simulink model "application"  (R2021b)
settings: Solver=FixedStepAuto  StartTime=0.0  StopTime=10.0  FixedStep=sampleTime  RelTol=1e-3
undefined symbols (not defined in the file or in its folder): AEMACE10_STBY, AEMACE8_STBY
libraries: simulink x10, EMACE_APP x6, AIL_STATE_MACHINE_LIB x2, AEMACE10_IN x1, AEMACE10_INSTRUMENTATION x1, AEMACE10_OUT x1, AEMACE8_IN x1, AEMACE8_INSTRUMENTATION x1, AEMACE8_OUT x1, SEMACE1_IN x1, SEMACE1_INSTRUMENTATION x1, SEMACE1_OUT x1
(part 1 of 2)
settings Model: Creator=ACH  LastModifiedBy=ACH

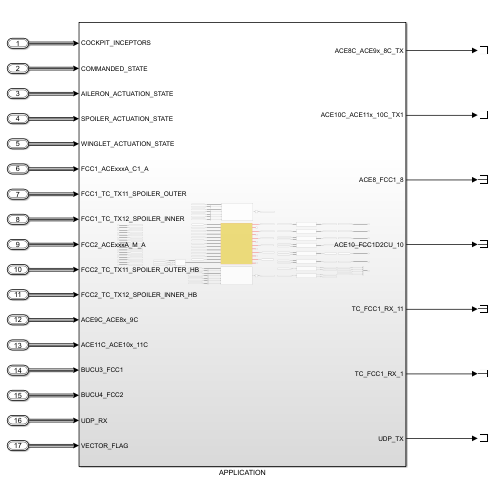
[thumbnail: Simulink's stored preview of the top-level diagram]
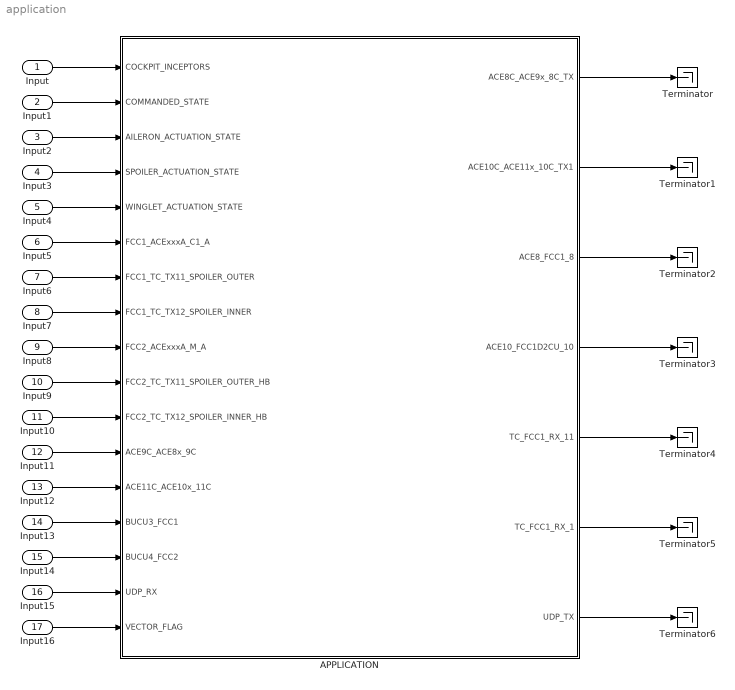
== system application ==
  Input : Inport  OutDataTypeStr=Bus: COCKPIT_INCEPTORS
  Input1 : Inport  Port=2  OutDataTypeStr=Bus: COMMANDED_STATE
  Input2 : Inport  Port=3  OutDataTypeStr=Bus: AILERON_ACTUATION_STATE
  Input3 : Inport  Port=4  OutDataTypeStr=Bus: SPOILER_ACTUATION_STATE
  Input4 : Inport  Port=5  OutDataTypeStr=Bus: WINGLET_ACTUATION_STATE
  Input5 : Inport  Port=6  OutDataTypeStr=Bus: FCC1_ACExxxA_C1_A
  Input6 : Inport  Port=7  OutDataTypeStr=Bus: FCC1_TC_TX_11_SPOILER_OUTER
  Input7 : Inport  Port=8  OutDataTypeStr=Bus: FCC1_TC_TX_12_SPOILER_INNER
  Input8 : Inport  Port=9  OutDataTypeStr=Bus: FCC2_ACExxxA_M_A
  Input9 : Inport  Port=10  OutDataTypeStr=Bus: FCC2_TC_TX_11_SPOILER_OUTER_HB
  Input10 : Inport  Port=11  OutDataTypeStr=Bus: FCC2_TC_TX_12_SPOILER_INNER_HB
  Input11 : Inport  Port=12  OutDataTypeStr=Bus: ACE9C_ACE8x_9C
  Input12 : Inport  Port=13  OutDataTypeStr=Bus: ACE11C_ACE10x_11C
  Input13 : Inport  Port=14  OutDataTypeStr=Bus: BUCU3_FCC1
  Input14 : Inport  Port=15  OutDataTypeStr=Bus: BUCU4_FCC2
  Input15 : Inport  Port=16  OutDataTypeStr=Bus: UDP_RX
  Input16 : Inport  Port=17  OutDataTypeStr=Bus: VECTOR_FLAG
  APPLICATION : Subsystem
  Terminator{,1..6} (7 alike) : Terminator
  wires:
  Input/1 -> APPLICATION/1(COCKPIT_INCEPTORS)
  Input1/1 -> APPLICATION/2(COMMANDED_STATE)
  Input2/1 -> APPLICATION/3(AILERON_ACTUATION_STATE)
  Input3/1 -> APPLICATION/4(SPOILER_ACTUATION_STATE)
  Input4/1 -> APPLICATION/5(WINGLET_ACTUATION_STATE)
  Input5/1 -> APPLICATION/6(FCC1_ACExxxA_C1_A)
  Input6/1 -> APPLICATION/7(FCC1_TC_TX11_SPOILER_OUTER)
  Input7/1 -> APPLICATION/8(FCC1_TC_TX12_SPOILER_INNER)
  Input8/1 -> APPLICATION/9(FCC2_ACExxxA_M_A)
  Input9/1 -> APPLICATION/10(FCC2_TC_TX11_SPOILER_OUTER_HB)
  Input10/1 -> APPLICATION/11(FCC2_TC_TX12_SPOILER_INNER_HB)
  Input11/1 -> APPLICATION/12(ACE9C_ACE8x_9C)
  Input12/1 -> APPLICATION/13(ACE11C_ACE10x_11C)
  Input13/1 -> APPLICATION/14(BUCU3_FCC1)
  Input14/1 -> APPLICATION/15(BUCU4_FCC2)
  Input15/1 -> APPLICATION/16(UDP_RX)
  Input16/1 -> APPLICATION/17(VECTOR_FLAG)
  APPLICATION/1(ACE8C_ACE9x_8C_TX) -> Terminator/1
  APPLICATION/2(ACE10C_ACE11x_10C_TX1) -> Terminator1/1
  APPLICATION/3(ACE8_FCC1_8) -> Terminator2/1
  APPLICATION/4(ACE10_FCC1D2CU_10) -> Terminator3/1
  APPLICATION/5(TC_FCC1_RX_11) -> Terminator4/1
  APPLICATION/6(TC_FCC1_RX_1) -> Terminator5/1
  APPLICATION/7(UDP_TX) -> Terminator6/1

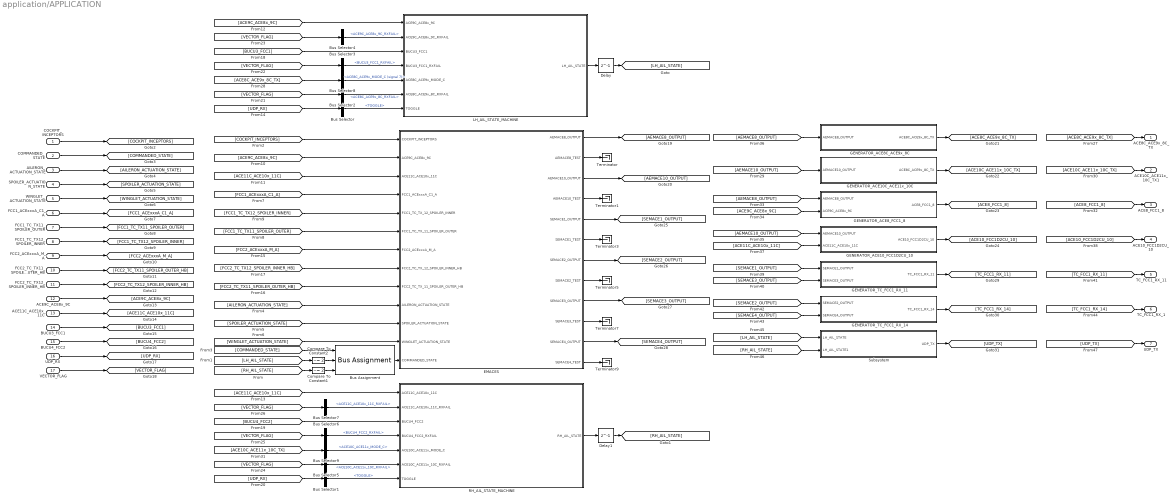
== system application/APPLICATION ==
  COCKPIT_INCEPTORS : Inport  OutDataTypeStr=Bus: COCKPIT_INCEPTORS
  COMMANDED_STATE : Inport  Port=2  OutDataTypeStr=Bus: COMMANDED_STATE
  AILERON_ACTUATION_STATE : Inport  Port=3  OutDataTypeStr=Bus: AILERON_ACTUATION_STATE
  SPOILER_ACTUATION_STATE : Inport  Port=4  OutDataTypeStr=Bus: SPOILER_ACTUATION_STATE
  WINGLET_ACTUATION_STATE : Inport  Port=5  OutDataTypeStr=Bus: WINGLET_ACTUATION_STATE
  FCC1_ACExxxA_C1_A : Inport  Port=6  OutDataTypeStr=Bus: FCC1_ACExxxA_C1_A
  FCC1_TC_TX11_SPOILER_OUTER : Inport  Port=7  OutDataTypeStr=Bus: FCC1_TC_TX_11_SPOILER_OUTER
  FCC1_TC_TX12_SPOILER_INNER : Inport  Port=8  OutDataTypeStr=Bus: FCC1_TC_TX_12_SPOILER_INNER
  FCC2_ACExxxA_M_A : Inport  Port=9  OutDataTypeStr=Bus: FCC2_ACExxxA_M_A
  FCC2_TC_TX11_SPOILER_OUTER_HB : Inport  Port=10  OutDataTypeStr=Bus: FCC2_TC_TX_11_SPOILER_OUTER_HB
  FCC2_TC_TX12_SPOILER_INNER_HB : Inport  Port=11  OutDataTypeStr=Bus: FCC2_TC_TX_12_SPOILER_INNER_HB
  ACE9C_ACE8x_9C : Inport  Port=12  OutDataTypeStr=Bus: ACE9C_ACE8x_9C
  ACE11C_ACE10x_11C : Inport  Port=13  OutDataTypeStr=Bus: ACE11C_ACE10x_11C
  BUCU3_FCC1 : Inport  Port=14  OutDataTypeStr=Bus: BUCU3_FCC1
  BUCU4_FCC2 : Inport  Port=15  OutDataTypeStr=Bus: BUCU4_FCC2
  UDP_RX : Inport  Port=16  OutDataTypeStr=Bus: UDP_RX
  VECTOR_FLAG : Inport  Port=17  OutDataTypeStr=Bus: VECTOR_FLAG
  Bus Assignment : BusAssignment  AssignedSignals=AEMACE8_STBY,AEMACE10_STBY
  Bus Selector : BusSelector  OutputSignals=TOGGLE
  Bus Selector1 : BusSelector  OutputSignals=TOGGLE
  Bus Selector2 : BusSelector  OutputSignals=ACE8C_ACE9x_8C_RXFAIL
  Bus Selector3 : BusSelector  OutputSignals=BUCU3_FCC1_RXFAIL
  Bus Selector4 : BusSelector  OutputSignals=ACE9C_ACE8x_9C_RXFAIL
  Bus Selector5 : BusSelector  OutputSignals=ACE10C_ACE11x_10C_RXFAIL
  Bus Selector6 : BusSelector  OutputSignals=BUCU4_FCC2_RXFAIL
  Bus Selector7 : BusSelector  OutputSignals=ACE11C_ACE10x_11C_RXFAIL
  Bus Selector8 : BusSelector  OutputSignals=ACE8C_ACE9x_MODE_C (signal 7)
  Bus Selector9 : BusSelector  OutputSignals=ACE10C_ACE11x_MODE_C
  Compare To Constant1 : simulink/Logic and Bit Operations/Compare To Constant  relop=~=  const=2  OutDataTypeStr=boolean
  Compare To Constant2 : simulink/Logic and Bit Operations/Compare To Constant  relop=~=  const=2  OutDataTypeStr=boolean
  Delay : Delay  DelayLength=1  InitialCondition=0
  Delay1 : Delay  DelayLength=1  InitialCondition=0
  EMACES : Subsystem
  GENERATOR_ACE10C_ACE11x_10C : Subsystem
  GENERATOR_ACE10_FCC1D2CU_10 : Subsystem
  GENERATOR_ACE8C_ACE9x_8C : Subsystem
  GENERATOR_ACE8_FCC1_8 : Subsystem
  GENERATOR_TC_FCC1_RX_11 : Subsystem
  GENERATOR_TC_FCC1_RX_14 : Subsystem
  LH_AIL_STATE_MACHINE : Subsystem
      settings: MinAlgLoopOccurrences=on
  RH_AIL_STATE_MACHINE : Subsystem
  Subsystem : Subsystem
  Terminator{,1,3,5,7,9} (6 alike) : Terminator
  ACE8C_ACE9x_8C_TX : Outport  OutDataTypeStr=Bus: ACE8C_ACE9x_8C
  ACE10C_ACE11x_10C_TX1 : Outport  Port=2  OutDataTypeStr=Bus: ACE10C_ACE11x_10C
  ACE8_FCC1_8 : Outport  Port=3  OutDataTypeStr=Bus: ACE8_FCC1_8
  ACE10_FCC1D2CU_10 : Outport  Port=4  OutDataTypeStr=Bus: ACE10_FCC1D2CU_10
  TC_FCC1_RX_11 : Outport  Port=5  OutDataTypeStr=Bus: TC_FCC1_RX_11
  TC_FCC1_RX_1 : Outport  Port=6  OutDataTypeStr=Bus: TC_FCC1_RX_14
  UDP_TX : Outport  Port=7  OutDataTypeStr=Bus: UDP_TX
  wires:
  [ACE11C_ACE10x_11C] -> EMACES/3(ACE11C_ACE10x_11C)
  [UDP_RX] -> Bus Selector1/1
  EMACES/9(SEMACE3_OUTPUT) -> [SEMACE3_OUTPUT]
  EMACES/12(SEMACE4_TEST) -> Terminator9/1
  Compare To Constant2/1 -> Bus Assignment/2
  RH_AIL_STATE_MACHINE/1(RH_AIL_STATE) -> Delay1/1
  [LH_AIL_STATE] -> Compare To Constant2/1
  [VECTOR_FLAG] -> Bus Selector4/1
  EMACES/11(SEMACE4_OUTPUT) -> [SEMACE4_OUTPUT]
  [AILERON_ACTUATION_STATE] -> EMACES/10(AILERON_ACTUATION_STATE)
  [ACE9C_ACE8x_9C] -> LH_AIL_STATE_MACHINE/1(ACE9C_ACE8x_9C)
  [ACE9C_ACE8x_9C] -> EMACES/2(ACE9C_ACE8x_9C)
  SPOILER_ACTUATION_STATE/1 -> [SPOILER_ACTUATION_STATE]
  [FCC2_ACExxxA_M_A] -> EMACES/7(FCC2_ACExxxA_M_A)
  Bus Selector1/1 -> RH_AIL_STATE_MACHINE/7(TOGGLE)  "<TOGGLE>"
  LH_AIL_STATE_MACHINE/1(LH_AIL_STATE) -> Delay/1
  Bus Selector2/1 -> LH_AIL_STATE_MACHINE/6(ACE8C_ACE9x_8C_RXFAIL)  "<ACE8C_ACE9x_8C_RXFAIL>"
  EMACES/6(SEMACE1_TEST) -> Terminator3/1
  EMACES/10(SEMACE3_TEST) -> Terminator7/1
  [WINGLET_ACTUATION_STATE] -> EMACES/12(WINGLET_ACTUATION_STATE)
  [FCC2_TC_TX11_SPOILER_OUTER_HB] -> EMACES/9(FCC2_TC_TX_11_SPOILER_OUTER_HB)
  [FCC1_ACExxxA_C1_A] -> EMACES/4(FCC1_ACExxxA_C1_A)
  [RH_AIL_STATE] -> Compare To Constant1/1
  WINGLET_ACTUATION_STATE/1 -> [WINGLET_ACTUATION_STATE]
  EMACES/5(SEMACE1_OUTPUT) -> [SEMACE1_OUTPUT]
  [SPOILER_ACTUATION_STATE] -> EMACES/11(SPOILER_ACTUATION_STATE)
  Bus Selector4/1 -> LH_AIL_STATE_MACHINE/2(ACE9C_ACE8x_9C_RXFAIL)  "<ACE9C_ACE8x_9C_RXFAIL>"
  BUCU3_FCC1/1 -> [BUCU3_FCC1]
  EMACES/2(AEMACE8_TEST) -> Terminator/1
  Bus Assignment/1 -> EMACES/13(COMMANDED_STATE)
  [COMMANDED_STATE] -> Bus Assignment/1
  FCC1_TC_TX11_SPOILER_OUTER/1 -> [FCC1_TC_TX11_SPOILER_OUTER]
  EMACES/4(AEMACE10_TEST) -> Terminator1/1
  EMACES/7(SEMACE2_OUTPUT) -> [SEMACE2_OUTPUT]
  [FCC1_TC_TX11_SPOILER_OUTER] -> EMACES/6(FCC1_TC_TX_11_SPOILER_OUTER)
  [UDP_RX] -> Bus Selector/1
  [VECTOR_FLAG] -> Bus Selector6/1
  Bus Selector7/1 -> RH_AIL_STATE_MACHINE/2(ACE11C_ACE10x_11C_RXFAIL)  "<ACE11C_ACE10x_11C_RXFAIL>"
  [VECTOR_FLAG] -> Bus Selector3/1
  Compare To Constant1/1 -> Bus Assignment/3
  Bus Selector3/1 -> LH_AIL_STATE_MACHINE/4(BUCU3_FCC1_RXFAIL)  "<BUCU3_FCC1_RXFAIL>"
  [VECTOR_FLAG] -> Bus Selector2/1
  [VECTOR_FLAG] -> Bus Selector5/1
  [FCC1_TC_TX12_SPOILER_INNER] -> EMACES/5(FCC1_TC_TX_12_SPOILER_INNER)
  Bus Selector/1 -> LH_AIL_STATE_MACHINE/7(TOGGLE)  "<TOGGLE>"
  Bus Selector5/1 -> RH_AIL_STATE_MACHINE/6(ACE10C_ACE11x_10C_RXFAIL)  "<ACE10C_ACE11x_10C_RXFAIL>"
  [BUCU4_FCC2] -> RH_AIL_STATE_MACHINE/3(BUCU4_FCC2)
  [ACE11C_ACE10x_11C] -> RH_AIL_STATE_MACHINE/1(ACE11C_ACE10x_11C)
  ACE11C_ACE10x_11C/1 -> [ACE11C_ACE10x_11C]
  EMACES/3(AEMACE10_OUTPUT) -> [AEMACE10_OUTPUT]
  [COCKPIT_INCEPTORS] -> EMACES/1(COCKPIT_INCEPTORS)
  Bus Selector6/1 -> RH_AIL_STATE_MACHINE/4(BUCU4_FCC2_RXFAIL)  "<BUCU4_FCC2_RXFAIL>"
  [FCC2_TC_TX12_SPOILER_INNER_HB] -> EMACES/8(FCC2_TC_TX_12_SPOILER_INNER_HB)
  EMACES/1(AEMACE8_OUTPUT) -> [AEMACE8_OUTPUT]
  FCC1_ACExxxA_C1_A/1 -> [FCC1_ACExxxA_C1_A]
  [VECTOR_FLAG] -> Bus Selector7/1
  [BUCU3_FCC1] -> LH_AIL_STATE_MACHINE/3(BUCU3_FCC1)
  EMACES/8(SEMACE2_TEST) -> Terminator5/1
  FCC2_ACExxxA_M_A/1 -> [FCC2_ACExxxA_M_A]
  COMMANDED_STATE/1 -> [COMMANDED_STATE]
  FCC2_TC_TX11_SPOILER_OUTER_HB/1 -> [FCC2_TC_TX11_SPOILER_OUTER_HB]
  ACE9C_ACE8x_9C/1 -> [ACE9C_ACE8x_9C]
  COCKPIT_INCEPTORS/1 -> [COCKPIT_INCEPTORS]
  UDP_RX/1 -> [UDP_RX]
  BUCU4_FCC2/1 -> [BUCU4_FCC2]
  FCC1_TC_TX12_SPOILER_INNER/1 -> [FCC1_TC_TX12_SPOILER_INNER]
  AILERON_ACTUATION_STATE/1 -> [AILERON_ACTUATION_STATE]
  FCC2_TC_TX12_SPOILER_INNER_HB/1 -> [FCC2_TC_TX12_SPOILER_INNER_HB]
  VECTOR_FLAG/1 -> [VECTOR_FLAG]
  Delay/1 -> [LH_AIL_STATE]
  Delay1/1 -> [RH_AIL_STATE]
  [ACE8C_ACE9x_8C_TX] -> ACE8C_ACE9x_8C_TX/1
  [AEMACE8_OUTPUT] -> GENERATOR_ACE8C_ACE9x_8C/1(AEMACE8_OUTPUT)
  GENERATOR_ACE8C_ACE9x_8C/1(ACE8C_ACE9x_8C_TX) -> [ACE8C_ACE9x_8C_TX]
  [ACE8C_ACE9x_8C_TX] -> Bus Selector8/1
  [AEMACE10_OUTPUT] -> GENERATOR_ACE10C_ACE11x_10C/1(AEMACE10_OUTPUT)
  GENERATOR_ACE10C_ACE11x_10C/1(ACE8C_ACE9x_8C_TX) -> [ACE10C_ACE11x_10C_TX]
  [ACE10C_ACE11x_10C_TX] -> ACE10C_ACE11x_10C_TX1/1
  [ACE10C_ACE11x_10C_TX] -> Bus Selector9/1
  Bus Selector9/1 -> RH_AIL_STATE_MACHINE/5(ACE10C_ACE11x_MODE_C)  "<ACE10C_ACE11x_MODE_C>"
  Bus Selector8/1 -> LH_AIL_STATE_MACHINE/5(ACE8C_ACE9x_MODE_C)  "<ACE8C_ACE9x_MODE_C (signal 7)>"
  GENERATOR_ACE8_FCC1_8/1(ACE8_FCC1_8) -> [ACE8_FCC1_8]
  [AEMACE8_OUTPUT] -> GENERATOR_ACE8_FCC1_8/1(AEMACE8_OUTPUT)
  [ACE8_FCC1_8] -> ACE8_FCC1_8/1
  [ACE9C_ACE8x_9C] -> GENERATOR_ACE8_FCC1_8/2(ACE9C_ACE8x_9C)
  [AEMACE10_OUTPUT] -> GENERATOR_ACE10_FCC1D2CU_10/1(AEMACE10_OUTPUT)
  [ACE11C_ACE10x_11C] -> GENERATOR_ACE10_FCC1D2CU_10/2(ACE11C_ACE10x_11C)
  GENERATOR_ACE10_FCC1D2CU_10/1(ACE10_FCC1D2CU_10) -> [ACE10_FCC1D2CU_10]
  [ACE10_FCC1D2CU_10] -> ACE10_FCC1D2CU_10/1
  [SEMACE1_OUTPUT] -> GENERATOR_TC_FCC1_RX_11/1(SEMACE1_OUTPUT)
  [SEMACE3_OUTPUT] -> GENERATOR_TC_FCC1_RX_11/2(SEMACE3_OUTPUT)
  GENERATOR_TC_FCC1_RX_11/1(TC_FCC1_RX_11) -> [TC_FCC1_RX_11]
  [TC_FCC1_RX_11] -> TC_FCC1_RX_11/1
  [TC_FCC1_RX_14] -> TC_FCC1_RX_1/1
  GENERATOR_TC_FCC1_RX_14/1(TC_FCC1_RX_14) -> [TC_FCC1_RX_14]
  [SEMACE4_OUTPUT] -> GENERATOR_TC_FCC1_RX_14/2(SEMACE4_OUTPUT)
  [SEMACE2_OUTPUT] -> GENERATOR_TC_FCC1_RX_14/1(SEMACE2_OUTPUT)
  [LH_AIL_STATE] -> Subsystem/1(LH_AIL_STATE)
  [RH_AIL_STATE] -> Subsystem/2(LH_AIL_STATE1)
  Subsystem/1(UDP_TX) -> [UDP_TX]
  [UDP_TX] -> UDP_TX/1

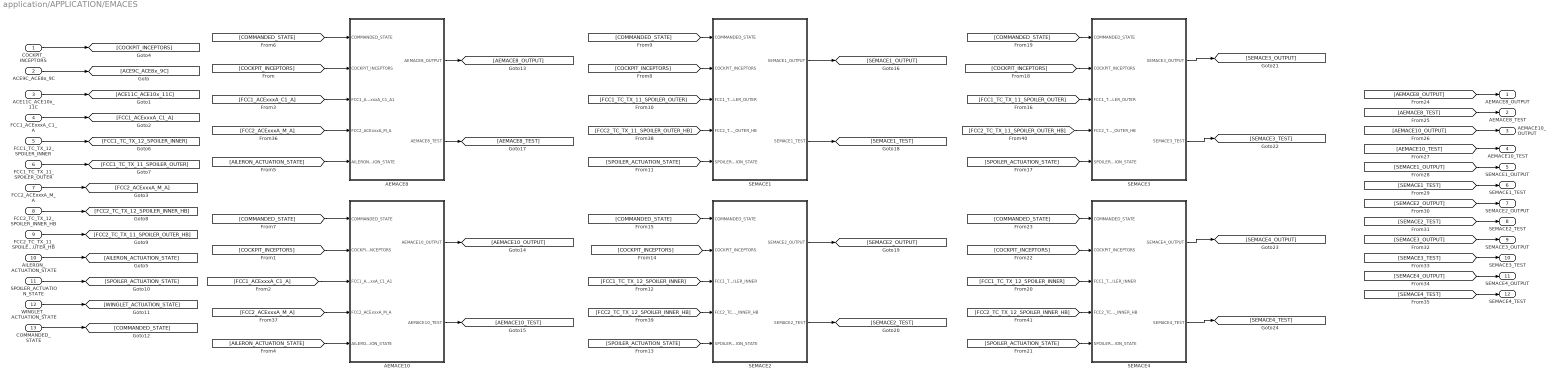
== system application/APPLICATION/EMACES ==
  COCKPIT_INCEPTORS : Inport  OutDataTypeStr=Bus: COCKPIT_INCEPTORS
  ACE9C_ACE8x_9C : Inport  Port=2  OutDataTypeStr=Bus: ACE9C_ACE8x_9C
  ACE11C_ACE10x_11C : Inport  Port=3  OutDataTypeStr=Bus: ACE11C_ACE10x_11C
  FCC1_ACExxxA_C1_A : Inport  Port=4  OutDataTypeStr=Bus: FCC1_ACExxxA_C1_A
  FCC1_TC_TX_12_SPOILER_INNER : Inport  Port=5  OutDataTypeStr=Bus: FCC1_TC_TX_12_SPOILER_INNER
  FCC1_TC_TX_11_SPOILER_OUTER : Inport  Port=6  OutDataTypeStr=Bus: FCC1_TC_TX_11_SPOILER_OUTER
  FCC2_ACExxxA_M_A : Inport  Port=7  OutDataTypeStr=Bus: FCC2_ACExxxA_M_A
  FCC2_TC_TX_12_SPOILER_INNER_HB : Inport  Port=8  OutDataTypeStr=Bus: FCC2_TC_TX_12_SPOILER_INNER_HB
  FCC2_TC_TX_11_SPOILER_OUTER_HB : Inport  Port=9  OutDataTypeStr=Bus: FCC2_TC_TX_11_SPOILER_OUTER_HB
  AILERON_ACTUATION_STATE : Inport  Port=10  OutDataTypeStr=Bus: AILERON_ACTUATION_STATE
  SPOILER_ACTUATION_STATE : Inport  Port=11  OutDataTypeStr=Bus: SPOILER_ACTUATION_STATE
  WINGLET_ACTUATION_STATE : Inport  Port=12  OutDataTypeStr=Bus: WINGLET_ACTUATION_STATE
  COMMANDED_STATE : Inport  Port=13  OutDataTypeStr=Bus: COMMANDED_STATE
  AEMACE10 : Subsystem
  AEMACE8 : Subsystem
  SEMACE1 : Subsystem
  SEMACE2 : Subsystem
  SEMACE3 : Subsystem
  SEMACE4 : Subsystem
  AEMACE8_OUTPUT : Outport  OutDataTypeStr=Bus: AEMACE8_OUTPUT
  AEMACE8_TEST : Outport  Port=2  OutDataTypeStr=Bus: AEMACE8_TEST
  AEMACE10_OUTPUT : Outport  Port=3  OutDataTypeStr=Bus: AEMACE10_OUTPUT
  AEMACE10_TEST : Outport  Port=4  OutDataTypeStr=Bus: AEMACE10_TEST
  SEMACE1_OUTPUT : Outport  Port=5  OutDataTypeStr=Bus: SEMACE1_OUTPUT
  SEMACE1_TEST : Outport  Port=6  OutDataTypeStr=Bus: SEMACE1_TEST
  SEMACE2_OUTPUT : Outport  Port=7  OutDataTypeStr=Bus: SEMACE3_OUTPUT
  SEMACE2_TEST : Outport  Port=8  OutDataTypeStr=Bus: SEMACE2_TEST
  SEMACE3_OUTPUT : Outport  Port=9  OutDataTypeStr=Bus: SEMACE3_OUTPUT
  SEMACE3_TEST : Outport  Port=10  OutDataTypeStr=Bus: SEMACE3_TEST
  SEMACE4_OUTPUT : Outport  Port=11  OutDataTypeStr=Bus: SEMACE4_OUTPUT
  SEMACE4_TEST : Outport  Port=12  OutDataTypeStr=Bus: SEMACE4_TEST
  wires:
  AEMACE8/1(AEMACE8_OUTPUT) -> [AEMACE8_OUTPUT]
  [SPOILER_ACTUATION_STATE] -> SEMACE4/5(SPOILER_ACTUATION_STATE)
  [AILERON_ACTUATION_STATE] -> AEMACE10/5(AILERON_ACTUATION_STATE)
  SEMACE2/1(SEMACE2_OUTPUT) -> [SEMACE2_OUTPUT]
  SEMACE4/2(SEMACE4_TEST) -> [SEMACE4_TEST]
  [COMMANDED_STATE] -> SEMACE1/1(COMMANDED_STATE)
  [FCC1_ACExxxA_C1_A] -> AEMACE8/3(FCC1_ACExxxA_C1_A1)
  AEMACE10/2(AEMACE10_TEST) -> [AEMACE10_TEST]
  [AEMACE8_OUTPUT] -> AEMACE8_OUTPUT/1
  SEMACE1/2(SEMACE1_TEST) -> [SEMACE1_TEST]
  AEMACE10/1(AEMACE10_OUTPUT) -> [AEMACE10_OUTPUT]
  [COMMANDED_STATE] -> AEMACE8/1(COMMANDED_STATE)
  SEMACE2/2(SEMACE2_TEST) -> [SEMACE2_TEST]
  [FCC1_TC_TX_11_SPOILER_OUTER] -> SEMACE1/3(FCC1_TC_TX_11_SPOILER_OUTER)
  ACE9C_ACE8x_9C/1 -> [ACE9C_ACE8x_9C]
  FCC1_TC_TX_11_SPOILER_OUTER/1 -> [FCC1_TC_TX_11_SPOILER_OUTER]
  [SPOILER_ACTUATION_STATE] -> SEMACE2/5(SPOILER_ACTUATION_STATE)
  [COMMANDED_STATE] -> SEMACE3/1(COMMANDED_STATE)
  AEMACE8/2(AEMACE8_TEST) -> [AEMACE8_TEST]
  [SEMACE3_OUTPUT] -> SEMACE3_OUTPUT/1
  [FCC1_ACExxxA_C1_A] -> AEMACE10/3(FCC1_ACExxxA_C1_A1)
  [AEMACE10_TEST] -> AEMACE10_TEST/1
  [COCKPIT_INCEPTORS] -> SEMACE1/2(COCKPIT_INCEPTORS)
  [AILERON_ACTUATION_STATE] -> AEMACE8/5(AILERON_ACTUATION_STATE)
  SEMACE1/1(SEMACE1_OUTPUT) -> [SEMACE1_OUTPUT]
  [COCKPIT_INCEPTORS] -> SEMACE2/2(COCKPIT_INCEPTORS)
  ACE11C_ACE10x_11C/1 -> [ACE11C_ACE10x_11C]
  [COCKPIT_INCEPTORS] -> SEMACE3/2(COCKPIT_INCEPTORS)
  [SEMACE1_OUTPUT] -> SEMACE1_OUTPUT/1
  [FCC1_TC_TX_12_SPOILER_INNER] -> SEMACE4/3(FCC1_TC_TX_12_SPOILER_INNER)
  FCC2_ACExxxA_M_A/1 -> [FCC2_ACExxxA_M_A]
  [COCKPIT_INCEPTORS] -> AEMACE8/2(COCKPIT_INCEPTORS)
  [COCKPIT_INCEPTORS] -> SEMACE4/2(COCKPIT_INCEPTORS)
  [AEMACE8_TEST] -> AEMACE8_TEST/1
  [FCC1_TC_TX_12_SPOILER_INNER] -> SEMACE2/3(FCC1_TC_TX_12_SPOILER_INNER)
  [SEMACE4_OUTPUT] -> SEMACE4_OUTPUT/1
  [COMMANDED_STATE] -> SEMACE2/1(COMMANDED_STATE)
  [FCC1_TC_TX_11_SPOILER_OUTER] -> SEMACE3/3(FCC1_TC_TX_11_SPOILER_OUTER)
  FCC1_ACExxxA_C1_A/1 -> [FCC1_ACExxxA_C1_A]
  [COMMANDED_STATE] -> SEMACE4/1(COMMANDED_STATE)
  [SEMACE1_TEST] -> SEMACE1_TEST/1
  SEMACE3/2(SEMACE3_TEST) -> [SEMACE3_TEST]
  SEMACE3/1(SEMACE3_OUTPUT) -> [SEMACE3_OUTPUT]
  [COMMANDED_STATE] -> AEMACE10/1(COMMANDED_STATE)
  COMMANDED_STATE/1 -> [COMMANDED_STATE]
  FCC1_TC_TX_12_SPOILER_INNER/1 -> [FCC1_TC_TX_12_SPOILER_INNER]
  [SPOILER_ACTUATION_STATE] -> SEMACE3/5(SPOILER_ACTUATION_STATE)
  [SPOILER_ACTUATION_STATE] -> SEMACE1/5(SPOILER_ACTUATION_STATE)
  SEMACE4/1(SEMACE4_OUTPUT) -> [SEMACE4_OUTPUT]
  [COCKPIT_INCEPTORS] -> AEMACE10/2(COCKPIT_INCEPTORS)
  [SEMACE2_OUTPUT] -> SEMACE2_OUTPUT/1
  [AEMACE10_OUTPUT] -> AEMACE10_OUTPUT/1
  AILERON_ACTUATION_STATE/1 -> [AILERON_ACTUATION_STATE]
  [SEMACE2_TEST] -> SEMACE2_TEST/1
  COCKPIT_INCEPTORS/1 -> [COCKPIT_INCEPTORS]
  FCC2_TC_TX_12_SPOILER_INNER_HB/1 -> [FCC2_TC_TX_12_SPOILER_INNER_HB]
  FCC2_TC_TX_11_SPOILER_OUTER_HB/1 -> [FCC2_TC_TX_11_SPOILER_OUTER_HB]
  WINGLET_ACTUATION_STATE/1 -> [WINGLET_ACTUATION_STATE]
  SPOILER_ACTUATION_STATE/1 -> [SPOILER_ACTUATION_STATE]
  [SEMACE3_TEST] -> SEMACE3_TEST/1
  [SEMACE4_TEST] -> SEMACE4_TEST/1
  [FCC2_ACExxxA_M_A] -> AEMACE8/4(FCC2_ACExxxA_M_A)
  [FCC2_ACExxxA_M_A] -> AEMACE10/4(FCC2_ACExxxA_M_A)
  [FCC2_TC_TX_11_SPOILER_OUTER_HB] -> SEMACE1/4(FCC2_TC_TX_11_SPOILER_OUTER_HB)
  [FCC2_TC_TX_12_SPOILER_INNER_HB] -> SEMACE2/4(FCC2_TC_TX_12_SPOILER_INNER_HB)
  [FCC2_TC_TX_11_SPOILER_OUTER_HB] -> SEMACE3/4(FCC2_TC_TX_11_SPOILER_OUTER_HB)
  [FCC2_TC_TX_12_SPOILER_INNER_HB] -> SEMACE4/4(FCC2_TC_TX_12_SPOILER_INNER_HB)

== system application/APPLICATION/GENERATOR_ACE10C_ACE11x_10C ==
  AEMACE10_OUTPUT : Inport  OutDataTypeStr=Bus: AEMACE10_OUTPUT
  Bus Creator : BusCreator  Inputs=17  OutDataTypeStr=Bus: ACE8C_ACE9x_8C
  Bus Selector8 : BusSelector  OutputSignals=AEMACE10_mode,AEMACE10_gearingAPP,AEMACE10_RAM_POS,AEMACE10_ROLL_POS,AEMACE10_SPD_SEL
  Cast{,2..10} (10 alike) : DataTypeConversion  OutDataTypeStr=boolean
  Cast1 : DataTypeConversion  OutDataTypeStr=uint8
  Cast11 : DataTypeConversion  OutDataTypeStr=single
  Constant{,1..11} (12 alike) : Constant  Value=0
  Delay{2..6} (5 alike) : Delay  DelayLength=1  InitialCondition=0
  ACE8C_ACE9x_8C_TX : Outport  OutDataTypeStr=Bus: ACE10C_ACE11x_10C
  wires:
  Bus Selector8/3 -> Delay4/1  "<AEMACE10_RAM_POS>"
  Bus Selector8/5 -> Delay6/1  "<AEMACE10_SPD_SEL>"
  Delay6/1 -> [ACE10C_ACE11x_SPD_C]
  AEMACE10_OUTPUT/1 -> Bus Selector8/1
  Delay5/1 -> [ACE10C_ACE11x_ROLL_POS_C]
  Constant7/1 -> Cast7/1
  Delay3/1 -> [ACE10C_ACE11x_GEARING_APPLIED]
  Cast10/1 -> Bus Creator/16
  Constant3/1 -> Cast3/1
  Cast11/1 -> Bus Creator/14
  [ACE10C_ACE11x_ROLL_POS_C] -> Bus Creator/9  "ACE10C_ACE11x_ROLL_POS_C"
  Cast5/1 -> Bus Creator/10
  [ACE10C_ACE11x_SPD_C] -> Bus Creator/17  "ACE10C_ACE11x_SPD_C"
  Constant8/1 -> Cast8/1
  Constant2/1 -> Cast2/1
  Bus Selector8/2 -> Delay3/1  "<AEMACE10_gearingAPP>"
  Cast3/1 -> Bus Creator/5
  Constant1/1 -> Cast1/1
  Constant5/1 -> Cast5/1
  Constant6/1 -> Cast6/1
  Bus Creator/1 -> ACE8C_ACE9x_8C_TX/1
  Cast1/1 -> Bus Creator/3
  Constant10/1 -> Cast10/1
  Delay2/1 -> [ACE10C_ACE11x_MODE_C]
  Cast6/1 -> Bus Creator/11
  Delay4/1 -> [ACE10C_ACE11x_RAM_POS_C]
  Cast8/1 -> Bus Creator/13
  Bus Selector8/4 -> Delay5/1  "<AEMACE10_ROLL_POS>"
  Constant11/1 -> Cast11/1
  Bus Selector8/1 -> Delay2/1  "<AEMACE10_mode>"
  Cast9/1 -> Bus Creator/15
  [ACE10C_ACE11x_GEARING_APPLIED] -> Bus Creator/1  "ACE10C_ACE11x_GEARING_APPLIED"
  Cast7/1 -> Bus Creator/12
  [ACE10C_ACE11x_RAM_POS_C] -> Bus Creator/6  "ACE10C_ACE11x_RAM_POS_C"
  Constant9/1 -> Cast9/1
  Constant/1 -> Cast/1
  Cast4/1 -> Bus Creator/8
  [ACE10C_ACE11x_MODE_C] -> Bus Creator/7  "ACE10C_ACE11x_MODE_C"
  Constant4/1 -> Cast4/1
  Cast2/1 -> Bus Creator/4
  Cast/1 -> Bus Creator/2  "ACE10C_ACE11x_GEARING_APP_F_C"

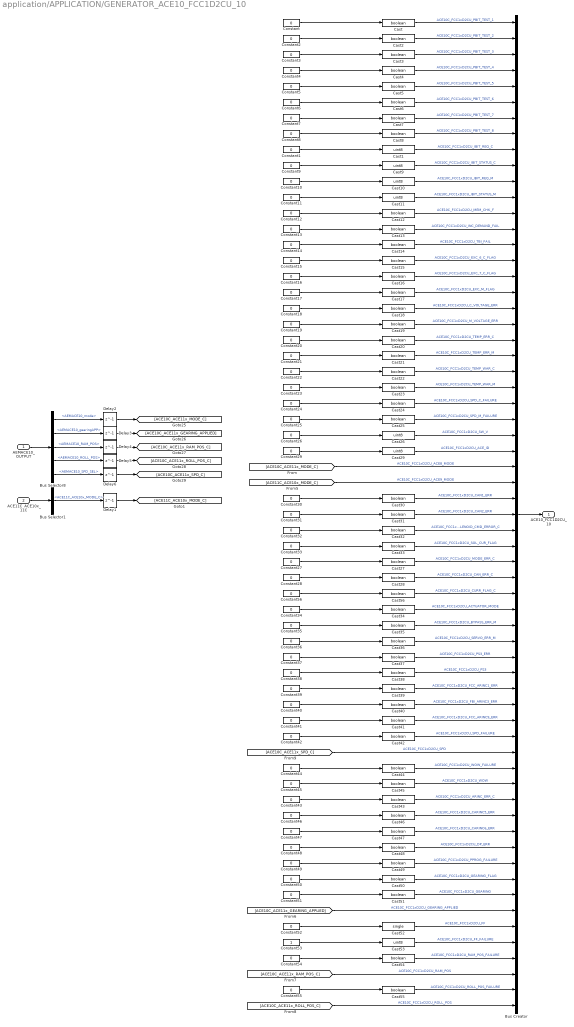
== system application/APPLICATION/GENERATOR_ACE10_FCC1D2CU_10 ==
  AEMACE10_OUTPUT : Inport  OutDataTypeStr=Bus: AEMACE10_OUTPUT
  ACE11C_ACE10x_11C : Inport  Port=2  OutDataTypeStr=Bus: ACE11C_ACE10x_11C
  Bus Creator : BusCreator  Inputs=63  OutDataTypeStr=Bus: ACE8_FCC1_8
  Bus Selector1 : BusSelector  OutputSignals=ACE11C_ACE10x_MODE_C
  Bus Selector8 : BusSelector  OutputSignals=AEMACE10_mode,AEMACE10_gearingAPP,AEMACE10_RAM_POS,AEMACE10_ROLL_POS,AEMACE10_SPD_SEL
  Cast{,2..8,12..25,27..28,30..51,54..56} (49 alike) : DataTypeConversion  OutDataTypeStr=boolean
  Cast{1,9..11,26,29,53} (7 alike) : DataTypeConversion  OutDataTypeStr=uint8
  Cast52 : DataTypeConversion  OutDataTypeStr=single
  Constant{,1..52,54..56} (56 alike) : Constant  Value=0
  Constant53 : Constant
  Delay{1..6} (6 alike) : Delay  DelayLength=1  InitialCondition=0
  ACE10_FCC1D2CU_10 : Outport  OutDataTypeStr=Bus: ACE10_FCC1D2CU_10
  wires:
  Cast56/1 -> Bus Creator/37  "ACE10C_FCC1xD2CU_CURR_FLAG_C"
  Constant56/1 -> Cast56/1
  Cast28/1 -> Bus Creator/36  "ACE10C_FCC1xD2CU_CAN_ERR_C"
  Constant28/1 -> Cast28/1
  Cast27/1 -> Bus Creator/35  "ACE10C_FCC1xD2CU_MODE_ERR_C"
  Constant27/1 -> Cast27/1
  Cast34/1 -> Bus Creator/38  "ACE10C_FCC1xD2CU_ACTUATOR_MODE"
  Cast36/1 -> Bus Creator/40  "ACE10C_FCC1xD2CU_SERVO_ERR_M"
  Constant34/1 -> Cast34/1
  Cast35/1 -> Bus Creator/39  "ACE10C_FCC1xD2CU_BYPASS_ERR_M"
  Constant36/1 -> Cast36/1
  Constant35/1 -> Cast35/1
  Constant39/1 -> Cast39/1
  Cast39/1 -> Bus Creator/43  "ACE10C_FCC1xD2CU_FCC_ARINC1_ERR"
  Cast37/1 -> Bus Creator/41  "ACE10C_FCC1xD2CU_PS3_ERR"
  Cast41/1 -> Bus Creator/45  "ACE10C_FCC1xD2CU_FCC_ARINC9_ERR"
  Constant38/1 -> Cast38/1
  Constant37/1 -> Cast37/1
  Cast38/1 -> Bus Creator/42  "ACE10C_FCC1xD2CU_PS3"
  Constant40/1 -> Cast40/1
  Constant41/1 -> Cast41/1
  Cast40/1 -> Bus Creator/44  "ACE10C_FCC1xD2CU_FBI_ARINC3_ERR"
  Cast44/1 -> Bus Creator/48  "ACE10C_FCC1xD2CU_WOW_FAILURE"
  Cast45/1 -> Bus Creator/49  "ACE10C_FCC1xD2CU_WOW"
  [ACE10C_ACE11x_SPD_C] -> Bus Creator/47  "ACE10C_FCC1xD2CU_SPD"
  Constant44/1 -> Cast44/1
  Cast42/1 -> Bus Creator/46  "ACE10C_FCC1xD2CU_SPD_FAILURE"
  Constant45/1 -> Cast45/1
  Constant42/1 -> Cast42/1
  Cast46/1 -> Bus Creator/51  "ACE10C_FCC1xD2CU_CARINC5_ERR"
  Cast48/1 -> Bus Creator/53  "ACE10C_FCC1xD2CU_DP_ERR"
  Constant48/1 -> Cast48/1
  Constant46/1 -> Cast46/1
  Cast43/1 -> Bus Creator/50  "ACE10C_FCC1xD2CU_ARINC_ERR_C"
  Constant43/1 -> Cast43/1
  Constant47/1 -> Cast47/1
  Cast47/1 -> Bus Creator/52  "ACE10C_FCC1xD2CU_CARINC6_ERR"
  Cast50/1 -> Bus Creator/55  "ACE10C_FCC1xD2CU_GEARING_FLAG"
  Cast51/1 -> Bus Creator/56  "ACE10C_FCC1xD2CU_GEARING"
  Cast49/1 -> Bus Creator/54  "ACE10C_FCC1xD2CU_PPROG_FAILURE"
  Constant50/1 -> Cast50/1
  Constant51/1 -> Cast51/1
  Constant49/1 -> Cast49/1
  [ACE10C_ACE11x_GEARING_APPLIED] -> Bus Creator/57  "ACE10C_FCC1xD2CU_GEARING_APPLIED"
  Constant53/1 -> Cast53/1
  Constant52/1 -> Cast52/1
  Cast52/1 -> Bus Creator/58  "ACE10C_FCC1xD2CU_FF"
  Cast53/1 -> Bus Creator/59  "ACE10C_FCC1xD2CU_FF_FAILURE"
  Cast54/1 -> Bus Creator/60  "ACE10C_FCC1xD2CU_RAM_POS_FAILURE"
  Constant54/1 -> Cast54/1
  [ACE10C_ACE11x_RAM_POS_C] -> Bus Creator/61  "ACE10C_FCC1xD2CU_RAM_POS"
  Constant55/1 -> Cast55/1
  Cast55/1 -> Bus Creator/62  "ACE10C_FCC1xD2CU_ROLL_POS_FAILURE"
  [ACE10C_ACE11x_ROLL_POS_C] -> Bus Creator/63  "ACE10C_FCC1xD2CU_ROLL_POS"
  [ACE11C_ACE10x_MODE_C] -> Bus Creator/30  "ACE10C_FCC1xD2CU_ACE9_MODE"
  Delay1/1 -> [ACE11C_ACE10x_MODE_C]
  Bus Selector1/1 -> Delay1/1  "<ACE11C_ACE10x_MODE_C>"
  ACE11C_ACE10x_11C/1 -> Bus Selector1/1
  Constant33/1 -> Cast33/1
  Cast33/1 -> Bus Creator/34  "ACE10C_FCC1xD2CU_SOL_CUR_FLAG"
  Cast32/1 -> Bus Creator/33  "ACE10C_FCC1xD2CU_SOLENOID_CMD_ERROR_C"
  Constant32/1 -> Cast32/1
  Constant31/1 -> Cast31/1
  Cast31/1 -> Bus Creator/32  "ACE10C_FCC1xD2CU_CAN2_ERR"
  Cast30/1 -> Bus Creator/31  "ACE10C_FCC1xD2CU_CAN1_ERR"
  Constant30/1 -> Cast30/1
  Cast26/1 -> Bus Creator/27  "ACE10C_FCC1xD2CU_SW_V"
  Constant26/1 -> Cast26/1
  Constant29/1 -> Cast29/1
  Cast29/1 -> Bus Creator/28  "ACE10C_FCC1xD2CU_ACE_ID"
  [ACE10C_ACE11x_MODE_C] -> Bus Creator/29  "ACE10C_FCC1xD2CU_ACE8_MODE"
  Constant25/1 -> Cast25/1
  Cast25/1 -> Bus Creator/26  "ACE10C_FCC1xD2CU_SPD_M_FAILURE"
  Cast24/1 -> Bus Creator/25  "ACE10C_FCC1xD2CU_SPD_C_FAILURE"
  Constant24/1 -> Cast24/1
  Constant23/1 -> Cast23/1
  Cast23/1 -> Bus Creator/24  "ACE10C_FCC1xD2CU_TEMP_WAR_M"
  Cast22/1 -> Bus Creator/23  "ACE10C_FCC1xD2CU_TEMP_WAR_C"
  Constant22/1 -> Cast22/1
  Constant21/1 -> Cast21/1
  Cast21/1 -> Bus Creator/22  "ACE10C_FCC1xD2CU_TEMP_ERR_M"
  Cast20/1 -> Bus Creator/21  "ACE10C_FCC1xD2CU_TEMP_ERR_C"
  Constant20/1 -> Cast20/1
  Constant19/1 -> Cast19/1
  Cast19/1 -> Bus Creator/20  "ACE10C_FCC1xD2CU_M_VOLTAGE_ERR"
  Cast18/1 -> Bus Creator/19  "ACE10C_FCC1xD2CU_C_VOLTAGE_ERR"
  Constant18/1 -> Cast18/1
  Constant17/1 -> Cast17/1
  Cast17/1 -> Bus Creator/18  "ACE10C_FCC1xD2CU_EXC_M_FLAG"
  Cast16/1 -> Bus Creator/17  "ACE10C_FCC1xD2CU_EXC_7_C_FLAG"
  Constant16/1 -> Cast16/1
  Constant15/1 -> Cast15/1
  Cast15/1 -> Bus Creator/16  "ACE10C_FCC1xD2CU_EXC_6_C_FLAG"
  Cast14/1 -> Bus Creator/15  "ACE10C_FCC1xD2CU_TBI_FAIL"
  Constant14/1 -> Cast14/1
  Constant13/1 -> Cast13/1
  Cast13/1 -> Bus Creator/14  "ACE10C_FCC1xD2CU_INC_DEMAND_FAIL"
  Cast12/1 -> Bus Creator/13  "ACE10C_FCC1xD2CU_MEM_CHK_F"
  Constant12/1 -> Cast12/1
  Cast11/1 -> Bus Creator/12  "ACE10C_FCC1xD2CU_IBIT_STATUS_M"
  Constant11/1 -> Cast11/1
  Constant10/1 -> Cast10/1
  Cast10/1 -> Bus Creator/11  "ACE10C_FCC1xD2CU_IBIT_REQ_M"
  Cast9/1 -> Bus Creator/10  "ACE10C_FCC1xD2CU_IBIT_STATUS_C"
  Constant9/1 -> Cast9/1
  Constant8/1 -> Cast8/1
  Cast8/1 -> Bus Creator/8  "ACE10C_FCC1xD2CU_PBIT_TEST_8"
  Cast7/1 -> Bus Creator/7  "ACE10C_FCC1xD2CU_PBIT_TEST_7"
  Constant7/1 -> Cast7/1
  Constant6/1 -> Cast6/1
  Cast6/1 -> Bus Creator/6  "ACE10C_FCC1xD2CU_PBIT_TEST_6"
  Cast5/1 -> Bus Creator/5  "ACE10C_FCC1xD2CU_PBIT_TEST_5"
  Constant5/1 -> Cast5/1
  Constant4/1 -> Cast4/1
  Cast4/1 -> Bus Creator/4  "ACE10C_FCC1xD2CU_PBIT_TEST_4"
  Cast3/1 -> Bus Creator/3  "ACE10C_FCC1xD2CU_PBIT_TEST_3"
  Constant3/1 -> Cast3/1
  Constant2/1 -> Cast2/1
  Cast2/1 -> Bus Creator/2  "ACE10C_FCC1xD2CU_PBIT_TEST_2"
  Constant1/1 -> Cast1/1
  Cast/1 -> Bus Creator/1  "ACE10C_FCC1xD2CU_PBIT_TEST_1"
  Constant/1 -> Cast/1
  Cast1/1 -> Bus Creator/9  "ACE10C_FCC1xD2CU_IBIT_REQ_C"
  Bus Selector8/1 -> Delay2/1  "<AEMACE10_mode>"
  Bus Selector8/4 -> Delay5/1  "<AEMACE10_ROLL_POS>"
  Delay4/1 -> [ACE10C_ACE11x_RAM_POS_C]
  Delay2/1 -> [ACE10C_ACE11x_MODE_C]
  Bus Creator/1 -> ACE10_FCC1D2CU_10/1
  Bus Selector8/2 -> Delay3/1  "<AEMACE10_gearingAPP>"
  Delay3/1 -> [ACE10C_ACE11x_GEARING_APPLIED]
  Delay5/1 -> [ACE10C_ACE11x_ROLL_POS_C]
  AEMACE10_OUTPUT/1 -> Bus Selector8/1
  Delay6/1 -> [ACE10C_ACE11x_SPD_C]
  Bus Selector8/5 -> Delay6/1  "<AEMACE10_SPD_SEL>"
  Bus Selector8/3 -> Delay4/1  "<AEMACE10_RAM_POS>"

== system application/APPLICATION/GENERATOR_ACE8C_ACE9x_8C ==
  AEMACE8_OUTPUT : Inport  OutDataTypeStr=Bus: AEMACE8_OUTPUT
  Bus Creator : BusCreator  Inputs=17  OutDataTypeStr=Bus: ACE8C_ACE9x_8C
  Bus Selector8 : BusSelector  OutputSignals=AEMACE8_mode,AEMACE8_gearingAPP,AEMACE8_RAM_POS,AEMACE8_ROLL_POS,AEMACE8_SPD_SEL
  Cast{,2..10} (10 alike) : DataTypeConversion  OutDataTypeStr=boolean
  Cast1 : DataTypeConversion  OutDataTypeStr=uint8
  Cast11 : DataTypeConversion  OutDataTypeStr=single
  Constant{,1..11} (12 alike) : Constant  Value=0
  Delay{2..6} (5 alike) : Delay  DelayLength=1  InitialCondition=0
  ACE8C_ACE9x_8C_TX : Outport  OutDataTypeStr=Bus: ACE8C_ACE9x_8C
  wires:
  Cast/1 -> Bus Creator/2  "ACE8C_ACE9x_GEARING_APP_F_C"
  Cast2/1 -> Bus Creator/4  "ACE8C_ACE9x_PPROG_FAILURE"
  Constant4/1 -> Cast4/1
  [ACE8C_ACE9x_MODE_C] -> Bus Creator/7  "ACE8C_ACE9x_MODE_C"
  Cast4/1 -> Bus Creator/8  "ACE8C_ACE9x_ROLL_POS_C_FAILURE"
  Constant/1 -> Cast/1
  Constant9/1 -> Cast9/1
  [ACE8C_ACE9x_RAM_POS_C] -> Bus Creator/6  "ACE8C_ACE9x_RAM_POS_C_FAILURE"
  Cast7/1 -> Bus Creator/12  "ACE8C_ACE9x_SPD_C_FAILURE"
  [ACE8C_ACE9x_GEARING_APPLIED] -> Bus Creator/1  "ACE8C_ACE9x_GEARING_APPLIED"
  Cast9/1 -> Bus Creator/15  "ACE8C_ACE9x_WOW1_C"
  Bus Selector8/1 -> Delay2/1  "<AEMACE8_mode>"
  Constant11/1 -> Cast11/1
  Bus Selector8/4 -> Delay5/1  "<AEMACE8_ROLL_POS>"
  Cast8/1 -> Bus Creator/13  "ACE8C_ACE9x_DELTA_P_FAILURE"
  Delay4/1 -> [ACE8C_ACE9x_RAM_POS_C]
  Cast6/1 -> Bus Creator/11  "ACE8C_ACE9x_TBI_FLAG_APP"
  Delay2/1 -> [ACE8C_ACE9x_MODE_C]
  Constant10/1 -> Cast10/1
  Cast1/1 -> Bus Creator/3  "ACE8C_ACE9x_PPROG"
  Bus Creator/1 -> ACE8C_ACE9x_8C_TX/1
  Constant6/1 -> Cast6/1
  Constant5/1 -> Cast5/1
  Constant1/1 -> Cast1/1
  Cast3/1 -> Bus Creator/5  "ACE8C_ACE9x_RAM_POS_C_FAILURE"
  Bus Selector8/2 -> Delay3/1  "<AEMACE8_gearingAPP>"
  Constant2/1 -> Cast2/1
  Constant8/1 -> Cast8/1
  [ACE8C_ACE9x_SPD_C] -> Bus Creator/17  "ACE8C_ACE9x_SPD_C"
  Cast5/1 -> Bus Creator/10  "ACE8C_ACE9x_INC_DEMAND_FAIL"
  [ACE8C_ACE9x_ROLL_POS_C] -> Bus Creator/9  "ACE8C_ACE9x_ROLL_POS_C"
  Cast11/1 -> Bus Creator/14  "ACE8C_ACE9x_DELTA_P_FAILURE"
  Constant3/1 -> Cast3/1
  Cast10/1 -> Bus Creator/16  "ACE8C_ACE9x_WOW2_C"
  Delay3/1 -> [ACE8C_ACE9x_GEARING_APPLIED]
  Constant7/1 -> Cast7/1
  Delay5/1 -> [ACE8C_ACE9x_ROLL_POS_C]
  AEMACE8_OUTPUT/1 -> Bus Selector8/1
  Delay6/1 -> [ACE8C_ACE9x_SPD_C]
  Bus Selector8/5 -> Delay6/1  "<AEMACE8_SPD_SEL>"
  Bus Selector8/3 -> Delay4/1  "<AEMACE8_RAM_POS>"

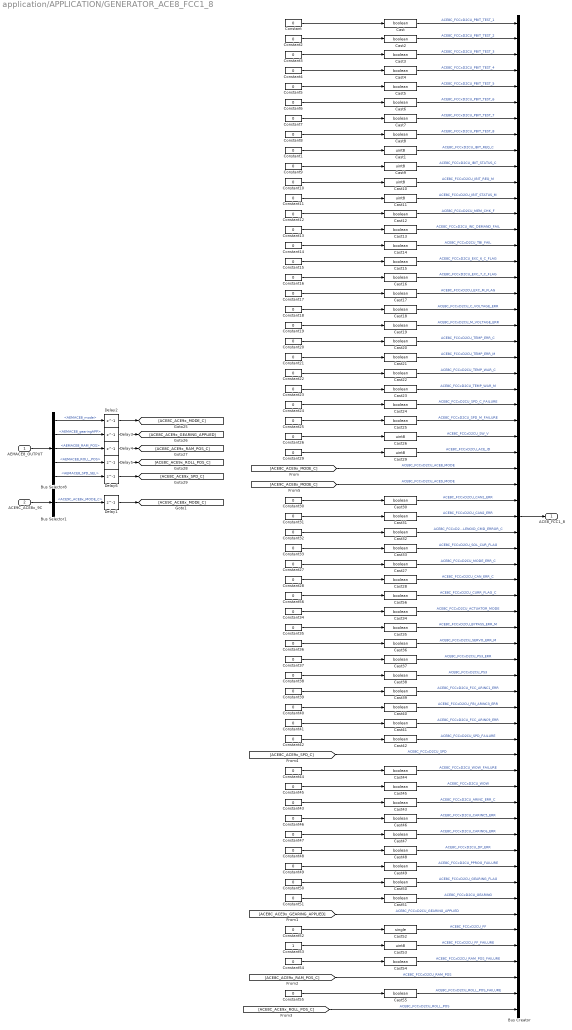
== system application/APPLICATION/GENERATOR_ACE8_FCC1_8 ==
  AEMACE8_OUTPUT : Inport  OutDataTypeStr=Bus: AEMACE8_OUTPUT
  ACE9C_ACE8x_9C : Inport  Port=2  OutDataTypeStr=Bus: ACE9C_ACE8x_9C
  Bus Creator : BusCreator  Inputs=63  OutDataTypeStr=Bus: ACE8_FCC1_8
  Bus Selector1 : BusSelector  OutputSignals=ACE9C_ACE8x_MODE_C
  Bus Selector8 : BusSelector  OutputSignals=AEMACE8_mode,AEMACE8_gearingAPP,AEMACE8_RAM_POS,AEMACE8_ROLL_POS,AEMACE8_SPD_SEL
  Cast{,2..8,12..25,27..28,30..51,54..56} (49 alike) : DataTypeConversion  OutDataTypeStr=boolean
  Cast{1,9..11,26,29,53} (7 alike) : DataTypeConversion  OutDataTypeStr=uint8
  Cast52 : DataTypeConversion  OutDataTypeStr=single
  Constant{,1..52,54..56} (56 alike) : Constant  Value=0
  Constant53 : Constant
  Delay{1..6} (6 alike) : Delay  DelayLength=1  InitialCondition=0
  ACE8_FCC1_8 : Outport  OutDataTypeStr=Bus: ACE8_FCC1_8
  wires:
  Bus Selector8/3 -> Delay4/1  "<AEMACE8_RAM_POS>"
  Bus Selector8/5 -> Delay6/1  "<AEMACE8_SPD_SEL>"
  Delay6/1 -> [ACE8C_ACE9x_SPD_C]
  AEMACE8_OUTPUT/1 -> Bus Selector8/1
  Delay5/1 -> [ACE8C_ACE9x_ROLL_POS_C]
  Delay3/1 -> [ACE8C_ACE9x_GEARING_APPLIED]
  Bus Selector8/2 -> Delay3/1  "<AEMACE8_gearingAPP>"
  Bus Creator/1 -> ACE8_FCC1_8/1
  Delay2/1 -> [ACE8C_ACE9x_MODE_C]
  Delay4/1 -> [ACE8C_ACE9x_RAM_POS_C]
  Bus Selector8/4 -> Delay5/1  "<AEMACE8_ROLL_POS>"
  Bus Selector8/1 -> Delay2/1  "<AEMACE8_mode>"
  Cast1/1 -> Bus Creator/9  "ACE8C_FCCxD2CU_IBIT_REQ_C"
  Constant/1 -> Cast/1
  Cast/1 -> Bus Creator/1  "ACE8C_FCCxD2CU_PBIT_TEST_1"
  Constant1/1 -> Cast1/1
  Cast2/1 -> Bus Creator/2  "ACE8C_FCCxD2CU_PBIT_TEST_2"
  Constant2/1 -> Cast2/1
  Constant3/1 -> Cast3/1
  Cast3/1 -> Bus Creator/3  "ACE8C_FCCxD2CU_PBIT_TEST_3"
  Cast4/1 -> Bus Creator/4  "ACE8C_FCCxD2CU_PBIT_TEST_4"
  Constant4/1 -> Cast4/1
  Constant5/1 -> Cast5/1
  Cast5/1 -> Bus Creator/5  "ACE8C_FCCxD2CU_PBIT_TEST_5"
  Cast6/1 -> Bus Creator/6  "ACE8C_FCCxD2CU_PBIT_TEST_6"
  Constant6/1 -> Cast6/1
  Constant7/1 -> Cast7/1
  Cast7/1 -> Bus Creator/7  "ACE8C_FCCxD2CU_PBIT_TEST_7"
  Cast8/1 -> Bus Creator/8  "ACE8C_FCCxD2CU_PBIT_TEST_8"
  Constant8/1 -> Cast8/1
  Constant9/1 -> Cast9/1
  Cast9/1 -> Bus Creator/10  "ACE8C_FCCxD2CU_IBIT_STATUS_C"
  Cast10/1 -> Bus Creator/11  "ACE8C_FCCxD2CU_IBIT_REQ_M"
  Constant10/1 -> Cast10/1
  Constant11/1 -> Cast11/1
  Cast11/1 -> Bus Creator/12  "ACE8C_FCCxD2CU_IBIT_STATUS_M"
  Constant12/1 -> Cast12/1
  Cast12/1 -> Bus Creator/13  "ACE8C_FCCxD2CU_MEM_CHK_F"
  Cast13/1 -> Bus Creator/14  "ACE8C_FCCxD2CU_INC_DEMAND_FAIL"
  Constant13/1 -> Cast13/1
  Constant14/1 -> Cast14/1
  Cast14/1 -> Bus Creator/15  "ACE8C_FCCxD2CU_TBI_FAIL"
  Cast15/1 -> Bus Creator/16  "ACE8C_FCCxD2CU_EXC_6_C_FLAG"
  Constant15/1 -> Cast15/1
  Constant16/1 -> Cast16/1
  Cast16/1 -> Bus Creator/17  "ACE8C_FCCxD2CU_EXC_7_C_FLAG"
  Cast17/1 -> Bus Creator/18  "ACE8C_FCCxD2CU_EXC_M_FLAG"
  Constant17/1 -> Cast17/1
  Constant18/1 -> Cast18/1
  Cast18/1 -> Bus Creator/19  "ACE8C_FCCxD2CU_C_VOLTAGE_ERR"
  Cast19/1 -> Bus Creator/20  "ACE8C_FCCxD2CU_M_VOLTAGE_ERR"
  Constant19/1 -> Cast19/1
  Constant20/1 -> Cast20/1
  Cast20/1 -> Bus Creator/21  "ACE8C_FCCxD2CU_TEMP_ERR_C"
  Cast21/1 -> Bus Creator/22  "ACE8C_FCCxD2CU_TEMP_ERR_M"
  Constant21/1 -> Cast21/1
  Constant22/1 -> Cast22/1
  Cast22/1 -> Bus Creator/23  "ACE8C_FCCxD2CU_TEMP_WAR_C"
  Cast23/1 -> Bus Creator/24  "ACE8C_FCCxD2CU_TEMP_WAR_M"
  Constant23/1 -> Cast23/1
  Constant24/1 -> Cast24/1
  Cast24/1 -> Bus Creator/25  "ACE8C_FCCxD2CU_SPD_C_FAILURE"
  Cast25/1 -> Bus Creator/26  "ACE8C_FCCxD2CU_SPD_M_FAILURE"
  Constant25/1 -> Cast25/1
  [ACE8C_ACE9x_MODE_C] -> Bus Creator/29  "ACE8C_FCCxD2CU_ACE8_MODE"
  Cast29/1 -> Bus Creator/28  "ACE8C_FCCxD2CU_ACE_ID"
  Constant29/1 -> Cast29/1
  Constant26/1 -> Cast26/1
  Cast26/1 -> Bus Creator/27  "ACE8C_FCCxD2CU_SW_V"
  Constant30/1 -> Cast30/1
  Cast30/1 -> Bus Creator/31  "ACE8C_FCCxD2CU_CAN1_ERR"
  Cast31/1 -> Bus Creator/32  "ACE8C_FCCxD2CU_CAN2_ERR"
  Constant31/1 -> Cast31/1
  Constant32/1 -> Cast32/1
  Cast32/1 -> Bus Creator/33  "ACE8C_FCCxD2CU_SOLENOID_CMD_ERROR_C"
  Cast33/1 -> Bus Creator/34  "ACE8C_FCCxD2CU_SOL_CUR_FLAG"
  Constant33/1 -> Cast33/1
  ACE9C_ACE8x_9C/1 -> Bus Selector1/1
  Bus Selector1/1 -> Delay1/1  "<ACE9C_ACE8x_MODE_C>"
  Delay1/1 -> [ACE9C_ACE8x_MODE_C]
  [ACE9C_ACE8x_MODE_C] -> Bus Creator/30  "ACE8C_FCCxD2CU_ACE9_MODE"
  [ACE8C_ACE9x_ROLL_POS_C] -> Bus Creator/63  "ACE8C_FCCxD2CU_ROLL_POS"
  Cast55/1 -> Bus Creator/62  "ACE8C_FCCxD2CU_ROLL_POS_FAILURE"
  Constant55/1 -> Cast55/1
  [ACE8C_ACE9x_RAM_POS_C] -> Bus Creator/61  "ACE8C_FCCxD2CU_RAM_POS"
  Constant54/1 -> Cast54/1
  Cast54/1 -> Bus Creator/60  "ACE8C_FCCxD2CU_RAM_POS_FAILURE"
  Cast53/1 -> Bus Creator/59  "ACE8C_FCCxD2CU_FF_FAILURE"
  Cast52/1 -> Bus Creator/58  "ACE8C_FCCxD2CU_FF"
  Constant52/1 -> Cast52/1
  Constant53/1 -> Cast53/1
  [ACE8C_ACE9x_GEARING_APPLIED] -> Bus Creator/57  "ACE8C_FCCxD2CU_GEARING_APPLIED"
  Constant49/1 -> Cast49/1
  Constant51/1 -> Cast51/1
  Constant50/1 -> Cast50/1
  Cast49/1 -> Bus Creator/54  "ACE8C_FCCxD2CU_PPROG_FAILURE"
  Cast51/1 -> Bus Creator/56  "ACE8C_FCCxD2CU_GEARING"
  Cast50/1 -> Bus Creator/55  "ACE8C_FCCxD2CU_GEARING_FLAG"
  Cast47/1 -> Bus Creator/52  "ACE8C_FCCxD2CU_CARINC6_ERR"
  Constant47/1 -> Cast47/1
  Constant43/1 -> Cast43/1
  Cast43/1 -> Bus Creator/50  "ACE8C_FCCxD2CU_ARINC_ERR_C"
  Constant46/1 -> Cast46/1
  Constant48/1 -> Cast48/1
  Cast48/1 -> Bus Creator/53  "ACE8C_FCCxD2CU_DP_ERR"
  Cast46/1 -> Bus Creator/51  "ACE8C_FCCxD2CU_CARINC5_ERR"
  Constant42/1 -> Cast42/1
  Constant45/1 -> Cast45/1
  Cast42/1 -> Bus Creator/46  "ACE8C_FCCxD2CU_SPD_FAILURE"
  Constant44/1 -> Cast44/1
  [ACE8C_ACE9x_SPD_C] -> Bus Creator/47  "ACE8C_FCCxD2CU_SPD"
  Cast45/1 -> Bus Creator/49  "ACE8C_FCCxD2CU_WOW"
  Cast44/1 -> Bus Creator/48  "ACE8C_FCCxD2CU_WOW_FAILURE"
  Cast40/1 -> Bus Creator/44  "ACE8C_FCCxD2CU_FBI_ARINC3_ERR"
  Constant41/1 -> Cast41/1
  Constant40/1 -> Cast40/1
  Cast38/1 -> Bus Creator/42  "ACE8C_FCCxD2CU_PS3"
  Constant37/1 -> Cast37/1
  Constant38/1 -> Cast38/1
  Cast41/1 -> Bus Creator/45  "ACE8C_FCCxD2CU_FCC_ARINC9_ERR"
  Cast37/1 -> Bus Creator/41  "ACE8C_FCCxD2CU_PS3_ERR"
  Cast39/1 -> Bus Creator/43  "ACE8C_FCCxD2CU_FCC_ARINC1_ERR"
  Constant39/1 -> Cast39/1
  Constant35/1 -> Cast35/1
  Constant36/1 -> Cast36/1
  Cast35/1 -> Bus Creator/39  "ACE8C_FCCxD2CU_BYPASS_ERR_M"
  Constant34/1 -> Cast34/1
  Cast36/1 -> Bus Creator/40  "ACE8C_FCCxD2CU_SERVO_ERR_M"
  Cast34/1 -> Bus Creator/38  "ACE8C_FCCxD2CU_ACTUATOR_MODE"
  Constant27/1 -> Cast27/1
  Cast27/1 -> Bus Creator/35  "ACE8C_FCCxD2CU_MODE_ERR_C"
  Constant28/1 -> Cast28/1
  Cast28/1 -> Bus Creator/36  "ACE8C_FCCxD2CU_CAN_ERR_C"
  Constant56/1 -> Cast56/1
  Cast56/1 -> Bus Creator/37  "ACE8C_FCCxD2CU_CURR_FLAG_C"

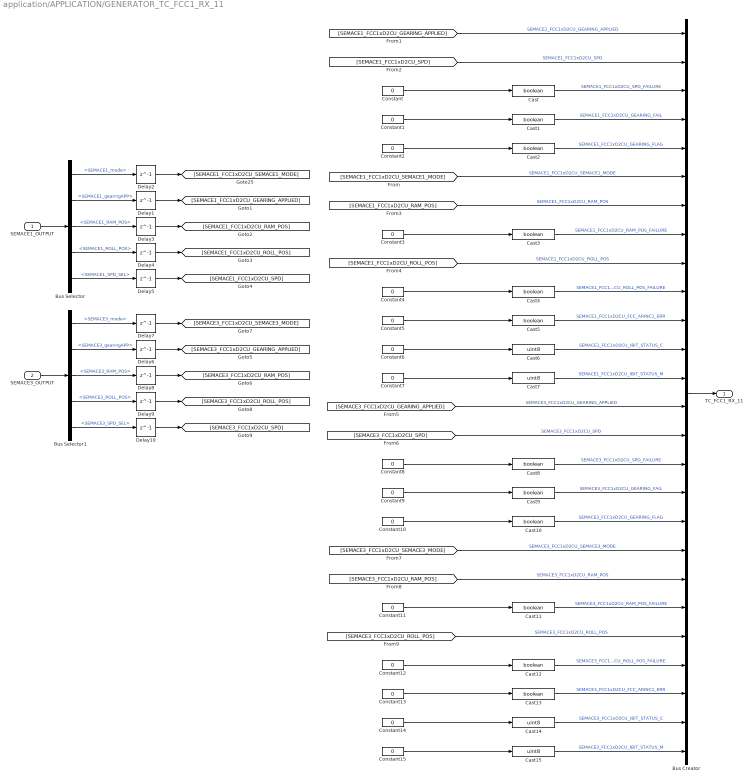
== system application/APPLICATION/GENERATOR_TC_FCC1_RX_11 ==
  SEMACE1_OUTPUT : Inport  OutDataTypeStr=Bus: SEMACE1_OUTPUT
  SEMACE3_OUTPUT : Inport  Port=2  OutDataTypeStr=Bus: SEMACE3_OUTPUT
  Bus Creator : BusCreator  Inputs=26  OutDataTypeStr=Bus: TC_FCC1_RX_11
  Bus Selector : BusSelector  OutputSignals=SEMACE1_mode,SEMACE1_gearingAPP,SEMACE1_RAM_POS,SEMACE1_ROLL_POS,SEMACE1_SPD_SEL
  Bus Selector1 : BusSelector  OutputSignals=SEMACE3_mode,SEMACE3_gearingAPP,SEMACE3_RAM_POS,SEMACE3_ROLL_POS,SEMACE3_SPD_SEL
  Cast{,1..5,8..13} (12 alike) : DataTypeConversion  OutDataTypeStr=boolean
  Cast{6..7,14..15} (4 alike) : DataTypeConversion  OutDataTypeStr=uint8
  Constant{,1..15} (16 alike) : Constant  Value=0
  Delay{1..10} (10 alike) : Delay  DelayLength=1  InitialCondition=0
  TC_FCC1_RX_11 : Outport  OutDataTypeStr=Bus: TC_FCC1_RX_11
  wires:
  SEMACE1_OUTPUT/1 -> Bus Selector/1
  SEMACE3_OUTPUT/1 -> Bus Selector1/1
  Delay2/1 -> [SEMACE1_FCC1xD2CU_SEMACE1_MODE]
  Bus Selector/1 -> Delay2/1  "<SEMACE1_mode>"
  Bus Selector/2 -> Delay1/1  "<SEMACE1_gearingAPP>"
  Delay1/1 -> [SEMACE1_FCC1xD2CU_GEARING_APPLIED]
  Delay3/1 -> [SEMACE1_FCC1xD2CU_RAM_POS]
  Bus Selector/3 -> Delay3/1  "<SEMACE1_RAM_POS>"
  Bus Selector/4 -> Delay4/1  "<SEMACE1_ROLL_POS>"
  Delay4/1 -> [SEMACE1_FCC1xD2CU_ROLL_POS]
  Delay5/1 -> [SEMACE1_FCC1xD2CU_SPD]
  Bus Selector/5 -> Delay5/1  "<SEMACE1_SPD_SEL>"
  Bus Selector1/5 -> Delay10/1  "<SEMACE3_SPD_SEL>"
  Delay10/1 -> [SEMACE3_FCC1xD2CU_SPD]
  Delay9/1 -> [SEMACE3_FCC1xD2CU_ROLL_POS]
  Bus Selector1/4 -> Delay9/1  "<SEMACE3_ROLL_POS>"
  Bus Selector1/3 -> Delay8/1  "<SEMACE3_RAM_POS>"
  Delay8/1 -> [SEMACE3_FCC1xD2CU_RAM_POS]
  Delay6/1 -> [SEMACE3_FCC1xD2CU_GEARING_APPLIED]
  Bus Selector1/2 -> Delay6/1  "<SEMACE3_gearingAPP>"
  Bus Selector1/1 -> Delay7/1  "<SEMACE3_mode>"
  Delay7/1 -> [SEMACE3_FCC1xD2CU_SEMACE3_MODE]
  Bus Creator/1 -> TC_FCC1_RX_11/1
  [SEMACE1_FCC1xD2CU_GEARING_APPLIED] -> Bus Creator/1  "SEMACE1_FCC1xD2CU_GEARING_APPLIED"
  [SEMACE1_FCC1xD2CU_SPD] -> Bus Creator/2  "SEMACE1_FCC1xD2CU_SPD"
  Cast/1 -> Bus Creator/3  "SEMACE1_FCC1xD2CU_SPD_FAILURE"
  Constant/1 -> Cast/1
  Constant1/1 -> Cast1/1
  Cast2/1 -> Bus Creator/5  "SEMACE1_FCC1xD2CU_GEARING_FLAG"
  Constant2/1 -> Cast2/1
  [SEMACE1_FCC1xD2CU_SEMACE1_MODE] -> Bus Creator/6  "SEMACE1_FCC1xD2CU_SEMACE1_MODE"
  [SEMACE1_FCC1xD2CU_RAM_POS] -> Bus Creator/7  "SEMACE1_FCC1xD2CU_RAM_POS"
  Constant3/1 -> Cast3/1
  Cast3/1 -> Bus Creator/8  "SEMACE1_FCC1xD2CU_RAM_POS_FAILURE"
  [SEMACE1_FCC1xD2CU_ROLL_POS] -> Bus Creator/9  "SEMACE1_FCC1xD2CU_ROLL_POS"
  Cast4/1 -> Bus Creator/10  "SEMACE1_FCC1xD2CU_ROLL_POS_FAILURE"
  Constant4/1 -> Cast4/1
  Constant5/1 -> Cast5/1
  Cast5/1 -> Bus Creator/11  "SEMACE1_FCC1xD2CU_FCC_ARINC1_ERR"
  Cast6/1 -> Bus Creator/12  "SEMACE1_FCC1xD2CU_IBIT_STATUS_C"
  Constant6/1 -> Cast6/1
  Constant7/1 -> Cast7/1
  Cast7/1 -> Bus Creator/13  "SEMACE1_FCC1xD2CU_IBIT_STATUS_M"
  Cast1/1 -> Bus Creator/4  "SEMACE1_FCC1xD2CU_GEARING_FAIL"
  [SEMACE3_FCC1xD2CU_GEARING_APPLIED] -> Bus Creator/14  "SEMACE3_FCC1xD2CU_GEARING_APPLIED"
  [SEMACE3_FCC1xD2CU_SPD] -> Bus Creator/15  "SEMACE3_FCC1xD2CU_SPD"
  Cast9/1 -> Bus Creator/17  "SEMACE3_FCC1xD2CU_GEARING_FAIL"
  Constant10/1 -> Cast10/1
  Cast10/1 -> Bus Creator/18  "SEMACE3_FCC1xD2CU_GEARING_FLAG"
  Constant9/1 -> Cast9/1
  Constant8/1 -> Cast8/1
  Cast8/1 -> Bus Creator/16  "SEMACE3_FCC1xD2CU_SPD_FAILURE"
  [SEMACE3_FCC1xD2CU_SEMACE3_MODE] -> Bus Creator/19  "SEMACE3_FCC1xD2CU_SEMACE3_MODE"
  [SEMACE3_FCC1xD2CU_RAM_POS] -> Bus Creator/20  "SEMACE3_FCC1xD2CU_RAM_POS"
  Cast11/1 -> Bus Creator/21  "SEMACE3_FCC1xD2CU_RAM_POS_FAILURE"
  Constant11/1 -> Cast11/1
  [SEMACE3_FCC1xD2CU_ROLL_POS] -> Bus Creator/22  "SEMACE3_FCC1xD2CU_ROLL_POS"
  Constant12/1 -> Cast12/1
  Cast12/1 -> Bus Creator/23  "SEMACE3_FCC1xD2CU_ROLL_POS_FAILURE"
  Cast13/1 -> Bus Creator/24  "SEMACE3_FCC1xD2CU_FCC_ARINC1_ERR"
  Constant13/1 -> Cast13/1
  Constant14/1 -> Cast14/1
  Cast14/1 -> Bus Creator/25  "SEMACE3_FCC1xD2CU_IBIT_STATUS_C"
  Constant15/1 -> Cast15/1
  Cast15/1 -> Bus Creator/26  "SEMACE3_FCC1xD2CU_IBIT_STATUS_M"

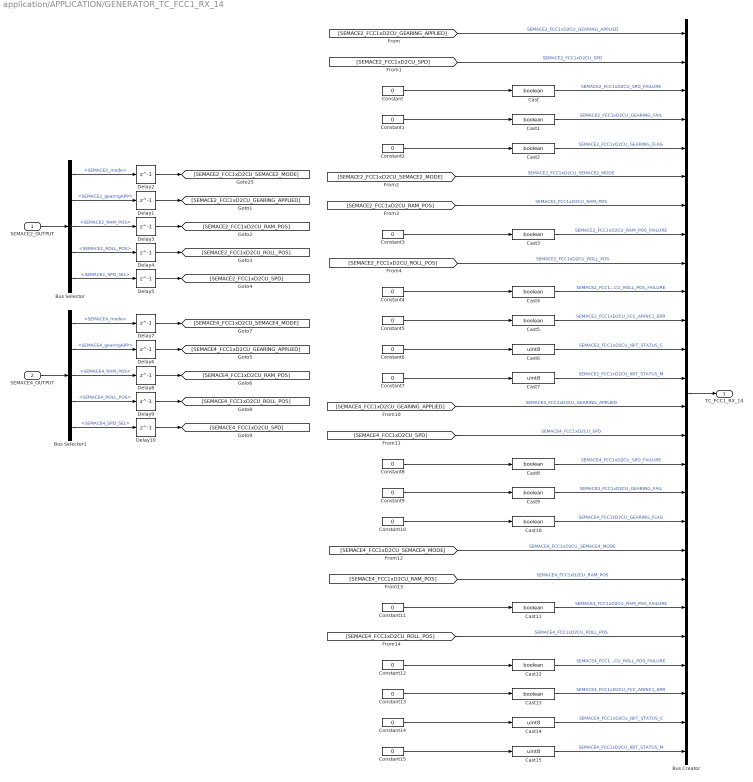
== system application/APPLICATION/GENERATOR_TC_FCC1_RX_14 ==
  SEMACE2_OUTPUT : Inport  OutDataTypeStr=Bus: SEMACE2_OUTPUT
  SEMACE4_OUTPUT : Inport  Port=2  OutDataTypeStr=Bus: SEMACE4_OUTPUT
  Bus Creator : BusCreator  Inputs=26  OutDataTypeStr=Bus: TC_FCC1_RX_11
  Bus Selector : BusSelector  OutputSignals=SEMACE2_mode,SEMACE2_gearingAPP,SEMACE2_RAM_POS,SEMACE2_ROLL_POS,SEMACE2_SPD_SEL
  Bus Selector1 : BusSelector  OutputSignals=SEMACE4_mode,SEMACE4_gearingAPP,SEMACE4_RAM_POS,SEMACE4_ROLL_POS,SEMACE4_SPD_SEL
  Cast{,1..5,8..13} (12 alike) : DataTypeConversion  OutDataTypeStr=boolean
  Cast{6..7,14..15} (4 alike) : DataTypeConversion  OutDataTypeStr=uint8
  Constant{,1..15} (16 alike) : Constant  Value=0
  Delay{1..10} (10 alike) : Delay  DelayLength=1  InitialCondition=0
  TC_FCC1_RX_14 : Outport  OutDataTypeStr=Bus: TC_FCC1_RX_14
  wires:
  Cast15/1 -> Bus Creator/26  "SEMACE4_FCC1xD2CU_IBIT_STATUS_M"
  Constant15/1 -> Cast15/1
  Cast14/1 -> Bus Creator/25  "SEMACE4_FCC1xD2CU_IBIT_STATUS_C"
  Constant14/1 -> Cast14/1
  Constant13/1 -> Cast13/1
  Cast13/1 -> Bus Creator/24  "SEMACE4_FCC1xD2CU_FCC_ARINC1_ERR"
  Cast12/1 -> Bus Creator/23  "SEMACE4_FCC1xD2CU_ROLL_POS_FAILURE"
  Constant12/1 -> Cast12/1
  [SEMACE4_FCC1xD2CU_ROLL_POS] -> Bus Creator/22  "SEMACE4_FCC1xD2CU_ROLL_POS"
  Constant11/1 -> Cast11/1
  Cast11/1 -> Bus Creator/21  "SEMACE4_FCC1xD2CU_RAM_POS_FAILURE"
  [SEMACE4_FCC1xD2CU_RAM_POS] -> Bus Creator/20  "SEMACE4_FCC1xD2CU_RAM_POS"
  [SEMACE4_FCC1xD2CU_SEMACE4_MODE] -> Bus Creator/19  "SEMACE4_FCC1xD2CU_SEMACE4_MODE"
  Cast8/1 -> Bus Creator/16  "SEMACE4_FCC1xD2CU_SPD_FAILURE"
  Constant8/1 -> Cast8/1
  Constant9/1 -> Cast9/1
  Cast10/1 -> Bus Creator/18  "SEMACE4_FCC1xD2CU_GEARING_FLAG"
  Constant10/1 -> Cast10/1
  Cast9/1 -> Bus Creator/17  "SEMACE4_FCC1xD2CU_GEARING_FAIL"
  [SEMACE4_FCC1xD2CU_SPD] -> Bus Creator/15  "SEMACE4_FCC1xD2CU_SPD"
  [SEMACE4_FCC1xD2CU_GEARING_APPLIED] -> Bus Creator/14  "SEMACE4_FCC1xD2CU_GEARING_APPLIED"
  Cast1/1 -> Bus Creator/4  "SEMACE2_FCC1xD2CU_GEARING_FAIL"
  Cast7/1 -> Bus Creator/13  "SEMACE2_FCC1xD2CU_IBIT_STATUS_M"
  Constant7/1 -> Cast7/1
  Constant6/1 -> Cast6/1
  Cast6/1 -> Bus Creator/12  "SEMACE2_FCC1xD2CU_IBIT_STATUS_C"
  Cast5/1 -> Bus Creator/11  "SEMACE2_FCC1xD2CU_FCC_ARINC1_ERR"
  Constant5/1 -> Cast5/1
  Constant4/1 -> Cast4/1
  Cast4/1 -> Bus Creator/10  "SEMACE2_FCC1xD2CU_ROLL_POS_FAILURE"
  [SEMACE2_FCC1xD2CU_ROLL_POS] -> Bus Creator/9  "SEMACE2_FCC1xD2CU_ROLL_POS"
  Cast3/1 -> Bus Creator/8  "SEMACE2_FCC1xD2CU_RAM_POS_FAILURE"
  Constant3/1 -> Cast3/1
  [SEMACE2_FCC1xD2CU_RAM_POS] -> Bus Creator/7  "SEMACE2_FCC1xD2CU_RAM_POS"
  [SEMACE2_FCC1xD2CU_SEMACE2_MODE] -> Bus Creator/6  "SEMACE2_FCC1xD2CU_SEMACE2_MODE"
  Constant2/1 -> Cast2/1
  Cast2/1 -> Bus Creator/5  "SEMACE2_FCC1xD2CU_GEARING_FLAG"
  Constant1/1 -> Cast1/1
  Constant/1 -> Cast/1
  Cast/1 -> Bus Creator/3  "SEMACE2_FCC1xD2CU_SPD_FAILURE"
  [SEMACE2_FCC1xD2CU_SPD] -> Bus Creator/2  "SEMACE2_FCC1xD2CU_SPD"
  [SEMACE2_FCC1xD2CU_GEARING_APPLIED] -> Bus Creator/1  "SEMACE2_FCC1xD2CU_GEARING_APPLIED"
  Bus Creator/1 -> TC_FCC1_RX_14/1
  Delay7/1 -> [SEMACE4_FCC1xD2CU_SEMACE4_MODE]
  Bus Selector1/1 -> Delay7/1  "<SEMACE4_mode>"
  Bus Selector1/2 -> Delay6/1  "<SEMACE4_gearingAPP>"
  Delay6/1 -> [SEMACE4_FCC1xD2CU_GEARING_APPLIED]
  Delay8/1 -> [SEMACE4_FCC1xD2CU_RAM_POS]
  Bus Selector1/3 -> Delay8/1  "<SEMACE4_RAM_POS>"
  Bus Selector1/4 -> Delay9/1  "<SEMACE4_ROLL_POS>"
  Delay9/1 -> [SEMACE4_FCC1xD2CU_ROLL_POS]
  Delay10/1 -> [SEMACE4_FCC1xD2CU_SPD]
  Bus Selector1/5 -> Delay10/1  "<SEMACE4_SPD_SEL>"
  Bus Selector/5 -> Delay5/1  "<SEMACE2_SPD_SEL>"
  Delay5/1 -> [SEMACE2_FCC1xD2CU_SPD]
  Delay4/1 -> [SEMACE2_FCC1xD2CU_ROLL_POS]
  Bus Selector/4 -> Delay4/1  "<SEMACE2_ROLL_POS>"
  Bus Selector/3 -> Delay3/1  "<SEMACE2_RAM_POS>"
  Delay3/1 -> [SEMACE2_FCC1xD2CU_RAM_POS]
  Delay1/1 -> [SEMACE2_FCC1xD2CU_GEARING_APPLIED]
  Bus Selector/2 -> Delay1/1  "<SEMACE2_gearingAPP>"
  Bus Selector/1 -> Delay2/1  "<SEMACE2_mode>"
  Delay2/1 -> [SEMACE2_FCC1xD2CU_SEMACE2_MODE]
  SEMACE4_OUTPUT/1 -> Bus Selector1/1
  SEMACE2_OUTPUT/1 -> Bus Selector/1

== system application/APPLICATION/LH_AIL_STATE_MACHINE ==
  ACE9C_ACE8x_9C : Inport  OutDataTypeStr=Bus: ACE9C_ACE8x_9C
  ACE9C_ACE8x_9C_RXFAIL : Inport  Port=2
  BUCU3_FCC1 : Inport  Port=3  OutDataTypeStr=Bus: BUCU3_FCC1
  BUCU3_FCC1_RXFAIL : Inport  Port=4
  ACE8C_ACE9x_MODE_C : Inport  Port=5
  ACE8C_ACE9x_8C_RXFAIL : Inport  Port=6
  TOGGLE : Inport  Port=7
  AILERON_STATE_MACHINE : AIL_STATE_MACHINE_LIB/AILERON_STATE_MACHINE  SystemSampleTime=-1  VariantActivationTime=update diagram  Latency=0  AutoFrameSizeCalculation=off
  LH_AIL_STATE_MACHINE_INPUT : LH_AIL_STATE_MACHINE_INPUT_LIB/LH_AIL_STATE_MACHINE_INPUT  SystemSampleTime=-1  VariantActivationTime=update diagram  Latency=0  AutoFrameSizeCalculation=off
  LH_AIL_STATE : Outport
  wires:
  AILERON_STATE_MACHINE/1 -> LH_AIL_STATE/1
  ACE9C_ACE8x_9C/1 -> LH_AIL_STATE_MACHINE_INPUT/1
  ACE9C_ACE8x_9C_RXFAIL/1 -> LH_AIL_STATE_MACHINE_INPUT/2
  BUCU3_FCC1/1 -> LH_AIL_STATE_MACHINE_INPUT/3
  BUCU3_FCC1_RXFAIL/1 -> LH_AIL_STATE_MACHINE_INPUT/4
  ACE8C_ACE9x_MODE_C/1 -> LH_AIL_STATE_MACHINE_INPUT/5
  ACE8C_ACE9x_8C_RXFAIL/1 -> LH_AIL_STATE_MACHINE_INPUT/6
  TOGGLE/1 -> LH_AIL_STATE_MACHINE_INPUT/7
  LH_AIL_STATE_MACHINE_INPUT/1 -> AILERON_STATE_MACHINE/1
  LH_AIL_STATE_MACHINE_INPUT/2 -> AILERON_STATE_MACHINE/2
  LH_AIL_STATE_MACHINE_INPUT/3 -> AILERON_STATE_MACHINE/3
  LH_AIL_STATE_MACHINE_INPUT/4 -> AILERON_STATE_MACHINE/4

== system application/APPLICATION/RH_AIL_STATE_MACHINE ==
  ACE11C_ACE10x_11C : Inport  OutDataTypeStr=Bus: ACE11C_ACE10x_11C
  ACE11C_ACE10x_11C_RXFAIL : Inport  Port=2
  BUCU4_FCC2 : Inport  Port=3  OutDataTypeStr=Bus: BUCU4_FCC2
  BUCU4_FCC2_RXFAIL : Inport  Port=4
  ACE10C_ACE11x_MODE_C : Inport  Port=5
  ACE10C_ACE11x_10C_RXFAIL : Inport  Port=6
  TOGGLE : Inport  Port=7
  AILERON_STATE_MACHINE : AIL_STATE_MACHINE_LIB/AILERON_STATE_MACHINE  SystemSampleTime=-1  VariantActivationTime=update diagram  Latency=0  AutoFrameSizeCalculation=off
  RH_AIL_STATE_MACHINE_INPUT : RH_AIL_STATE_MACHINE_INPUT_LIB/RH_AIL_STATE_MACHINE_INPUT  SystemSampleTime=-1  VariantActivationTime=update diagram  Latency=0  AutoFrameSizeCalculation=off
  RH_AIL_STATE : Outport
  wires:
  ACE11C_ACE10x_11C_RXFAIL/1 -> RH_AIL_STATE_MACHINE_INPUT/2
  BUCU4_FCC2/1 -> RH_AIL_STATE_MACHINE_INPUT/3
  RH_AIL_STATE_MACHINE_INPUT/1 -> AILERON_STATE_MACHINE/1
  RH_AIL_STATE_MACHINE_INPUT/4 -> AILERON_STATE_MACHINE/4
  RH_AIL_STATE_MACHINE_INPUT/3 -> AILERON_STATE_MACHINE/3
  AILERON_STATE_MACHINE/1 -> RH_AIL_STATE/1
  RH_AIL_STATE_MACHINE_INPUT/2 -> AILERON_STATE_MACHINE/2
  ACE11C_ACE10x_11C/1 -> RH_AIL_STATE_MACHINE_INPUT/1
  ACE10C_ACE11x_10C_RXFAIL/1 -> RH_AIL_STATE_MACHINE_INPUT/6
  TOGGLE/1 -> RH_AIL_STATE_MACHINE_INPUT/7
  BUCU4_FCC2_RXFAIL/1 -> RH_AIL_STATE_MACHINE_INPUT/4
  ACE10C_ACE11x_MODE_C/1 -> RH_AIL_STATE_MACHINE_INPUT/5

== system application/APPLICATION/Subsystem ==
  LH_AIL_STATE : Inport
  LH_AIL_STATE1 : Inport  Port=2
  Bus Creator : BusCreator  Inputs=4  OutDataTypeStr=Bus: UDP_TX
  GENERATOR_STATE_CMD_LH_AIL : Subsystem
  GENERATOR_STATE_CMD_RH_AIL : Subsystem
  UDP_TX : Outport  OutDataTypeStr=Bus: UDP_TX
  wires:
  GENERATOR_STATE_CMD_RH_AIL/2(ACE11_CMD_STATE) -> [ACE11_CMD_STATE]
  [AEMACE10_CMD_STATE] -> Bus Creator/3  "AEMACE10_CMD_STATE"
  GENERATOR_STATE_CMD_LH_AIL/1(AEMACE8_CMD_STATE) -> [AEMACE8_CMD_STATE]
  [ACE9_CMD_STATE] -> Bus Creator/2  "ACE9_CMD_STATE"
  [AEMACE8_CMD_STATE] -> Bus Creator/1  "AEMACE8_CMD_STATE"
  GENERATOR_STATE_CMD_LH_AIL/2(ACE9_CMD_STATE) -> [ACE9_CMD_STATE]
  GENERATOR_STATE_CMD_RH_AIL/1(AEMACE10_CMD_STATE) -> [AEMACE10_CMD_STATE]
  LH_AIL_STATE1/1 -> GENERATOR_STATE_CMD_RH_AIL/1(LH_AIL_STATE)
  [ACE11_CMD_STATE] -> Bus Creator/4  "ACE11_CMD_STATE"
  LH_AIL_STATE/1 -> GENERATOR_STATE_CMD_LH_AIL/1(LH_AIL_STATE)
  Bus Creator/1 -> UDP_TX/1
